simulink model "IdealFixedGearTransmissionSSC"  (R2026b)
settings: Solver=VariableStepAuto
undefined symbols (not defined in the file): Diff, Eng, PlntTransDampVect, Trans
libraries: fl_lib x6, nesl_utility x4, nesl_utility_internal x1, sdl_lib x1
settings Model: ModifiedByFormat=The MathWorks, Inc.  Creator=The MathWorks, Inc.  LastModifiedBy=The MathWorks, Inc.
settings OptimizationCC: ReuseModelBlockBuffer=off
settings DebuggingCC: SubsystemReferenceDiagnosticForUnitTest=warning
settings SimscapeCC: SimscapeUseEnergyAccounting=off

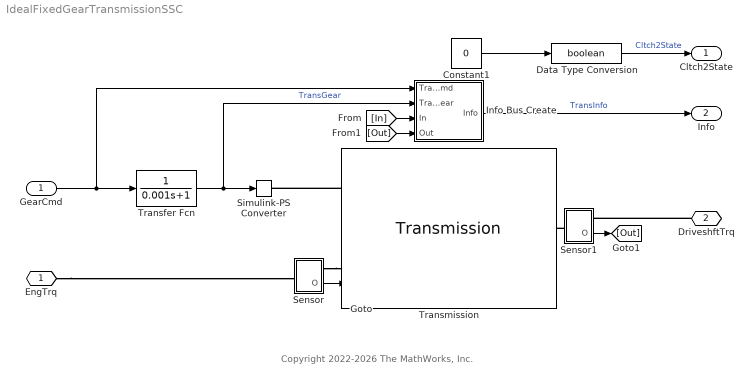
== system IdealFixedGearTransmissionSSC ==
  note: Copyright 2022-2026 The MathWorks, Inc.
  GearCmd : Inport
  Constant1 : Constant  Value=0  SampleTime=-1
  Data Type Conversion : DataTypeConversion  OutDataTypeStr=boolean  SaturateOnIntegerOverflow=off  RndMeth=Floor
  Info Bus Create : Subsystem
  Sensor : Subsystem
      settings: PortSchema="{\"entries\":[{\"content\":{\"sides\":[{\"content\":{\"connectorIds\":[\"LConn1\"]},\"type\":\"ConnectorPlacement.EquallySpacedRectSide\",\"uuid\":\"2e27b447-89d7-4d94-b9d2-8f612a4e25ed\"},{\"content\":{\"connectorIds\":[\"RConn1\",\"Out1\"],\"side\":\"RIGHT\"},\"type\":\"ConnectorPlacement.EquallySpacedRectSide\",\"uuid\":\"d649ff29-a00c-460e-9e09-fe3bc3dd9339\"},{\"content\":{\"side\":\"TOP\"},\"type\":\"ConnectorPlacement.EquallySpacedRectSide\",\"uuid\":\"c1caa1bf-44c8-4179-bd35-f8aecae525f1\"}]},\"type\":\"ConnectorPlacement.EquallySpacedConnector\",\"uuid\":\"741ea5ec-6556-46e5-ba1b-80e523f861d6\"}],\"packageUris\":[\"http://schema.mathworks.com/mf0/Connector/R2020b\"],\"version\":\"1.0\"}"
  Sensor1 : Subsystem
      settings: PortSchema="{\"entries\":[{\"content\":{\"sides\":[{\"content\":{\"connectorIds\":[\"LConn1\"]},\"type\":\"ConnectorPlacement.EquallySpacedRectSide\",\"uuid\":\"2e27b447-89d7-4d94-b9d2-8f612a4e25ed\"},{\"content\":{\"connectorIds\":[\"RConn1\",\"Out1\"],\"side\":\"RIGHT\"},\"type\":\"ConnectorPlacement.EquallySpacedRectSide\",\"uuid\":\"d649ff29-a00c-460e-9e09-fe3bc3dd9339\"},{\"content\":{\"side\":\"TOP\"},\"type\":\"ConnectorPlacement.EquallySpacedRectSide\",\"uuid\":\"c1caa1bf-44c8-4179-bd35-f8aecae525f1\"}]},\"type\":\"ConnectorPlacement.EquallySpacedConnector\",\"uuid\":\"741ea5ec-6556-46e5-ba1b-80e523f861d6\"}],\"packageUris\":[\"http://schema.mathworks.com/mf0/Connector/R2020b\"],\"version\":\"1.0\"}"
  Simulink-PS Converter : nesl_utility_internal/Simulink-PS Converter  PhysicalDomain=network_engine_domain  SubClassName=ps_input  LeftPortType=input  RightPortType=output  PseudoPeriodic=off  Frequencies=[]  NoiseDistribution=none  NoiseParameters=[]  Unit=1  AffineConversion=off  FilteringAndDerivatives=provide  SimscapeFilterOrder=1  InputFilterTimeConstant=0.001  UdotUserProvided=0
  Transfer Fcn : TransferFcn  Denominator=[0.001 1]
  Transmission : sdl_lib/Gears/Transmission  gear_ratios=PlntTransGearRatioVect(3:end)  reverse_ratio=PlntTransRvrseGearRatio  friction_model=sdl.enum.transmissionFriction.gear  efficiency=0.95  efficiency_tlu=PlntTransEffVect(3:end)  reverse_efficiency=PlntTransRvrseGearEff  pwr_thr=PlntTransPwrThresh W  kp=PlntTransStiff N*m/rad  kv=PlntTransDamp N*m*s/rad  initial_torque=PlntTransInitInTrq N*m  mu_visc=[PlntTransDampVect(2), PlntTransDampVect(2)] N*m*s/rad  t_friction=PlntTransCltchKinFricTrq N*m  t_locked=PlntTransCltchStatFricTrq N*m  shift_model=sdl.enum.transmissionShiftModel.instant  shift_time=PlntTransCltchShiftTime ms  w_tol=PlntTransCltchVelTol rad/s  initial_state_locked=sdl.enum.initial_lock.locked  thermal_port=simscape.enum.thermaleffects.omit  thermal_mass=100 kJ/K  initial_temperature=300 K
      settings: LogSimulationData=on
  EngTrq : PMIOPort  Side=Left
  DriveshftTrq : PMIOPort  Port=2  Side=Right
  Cltch2State : Outport  VectorParamsAs1DForOutWhenUnconnected=off
  Info : Outport  Port=2  VectorParamsAs1DForOutWhenUnconnected=off
  wires:
  Sensor1/1(O) -> [Out]
  Sensor/1(O) -> [In]
  Info Bus Create/1(Info) -> Info/1  "TransInfo"
  [Out] -> Info Bus Create/4(Out)
  [In] -> Info Bus Create/3(In)
  GearCmd/1 -> Transfer Fcn/1, Info Bus Create/1(TransGearCmd)
  Transfer Fcn/1 -> Simulink-PS Converter/1, Info Bus Create/2(TransGear)  "TransGear"
  Constant1/1 -> Data Type Conversion/1
  Data Type Conversion/1 -> Cltch2State/1  "Cltch2State"
  connections:
  Sensor1/LConn1 -- Transmission/RConn1
  Sensor/RConn1 -- Transmission/LConn2
  DriveshftTrq/RConn1 -- Sensor1/RConn1
  EngTrq/RConn1 -- Sensor/LConn1
  Transmission/LConn1 -- Simulink-PS Converter/RConn1

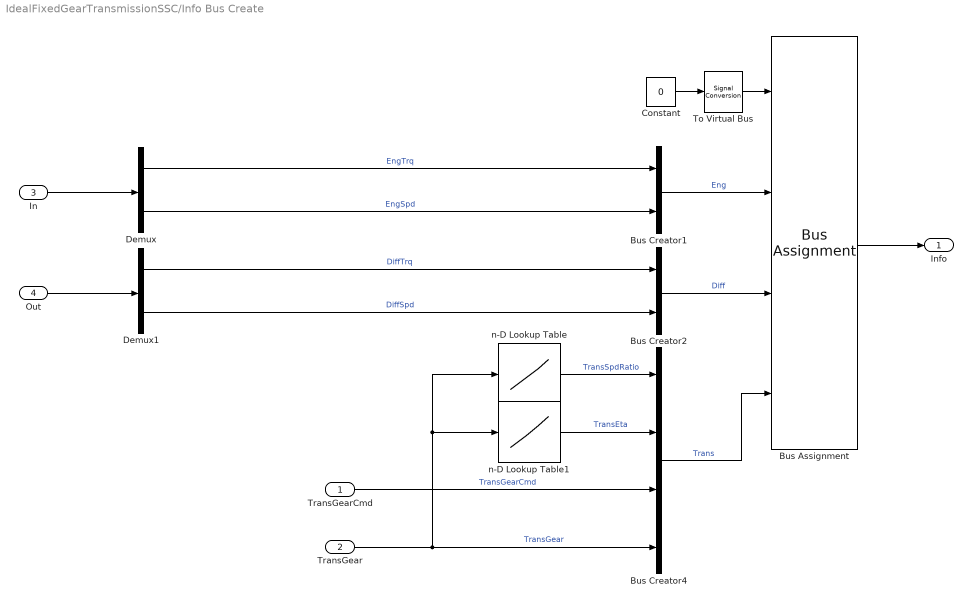
== system IdealFixedGearTransmissionSSC/Info Bus Create ==
  TransGearCmd : Inport
  TransGear : Inport  Port=2
  In : Inport  Port=3
  Out : Inport  Port=4
  Bus Assignment : BusAssignment  AssignedSignals=Eng,Diff,Trans
  Bus Creator1 : BusCreator  Inputs=2
  Bus Creator2 : BusCreator  Inputs=2
  Bus Creator4 : BusCreator  Inputs=4
  Constant : Constant  Value=0  OutDataTypeStr=Bus: InfoBUS  SampleTime=Inf
  Demux : Demux  Outputs=2
  Demux1 : Demux  Outputs=2
  To Virtual Bus : SignalConversion  ConversionOutput=Virtual bus  OverrideOpt=off
  n-D Lookup Table : Lookup_n-D  NumberOfTableDimensions=1  BreakpointsForDimension1=PlntTransGearNumVect(2:end)  BreakpointsForDimension3=[5, 7]  BeginIndexSearchUsingPreviousIndexResult=on  Table=PlntTransGearRatioVect(2:end)  InterpMethod=Nearest  ExtrapMethod=Clip  UseLastTableValue=on  InternalRulePriority=Speed  RndMeth=Simplest
  n-D Lookup Table1 : Lookup_n-D  NumberOfTableDimensions=1  BreakpointsForDimension1=PlntTransGearNumVect(2:end)  BreakpointsForDimension3=[5, 7]  BeginIndexSearchUsingPreviousIndexResult=on  Table=PlntTransEffVect(2:end)  InterpMethod=Nearest  ExtrapMethod=Clip  UseLastTableValue=on  InternalRulePriority=Speed  RndMeth=Simplest
  Info : Outport
  wires:
  To Virtual Bus/1 -> Bus Assignment/1
  Bus Assignment/1 -> Info/1
  Constant/1 -> To Virtual Bus/1
  Bus Creator2/1 -> Bus Assignment/3  "Diff"
  TransGear/1 -> Bus Creator4/4, n-D Lookup Table1/1, n-D Lookup Table/1  "TransGear"
  Demux/1 -> Bus Creator1/1  "EngTrq"
  n-D Lookup Table/1 -> Bus Creator4/1  "TransSpdRatio"
  Demux1/1 -> Bus Creator2/1  "DiffTrq"
  Demux/2 -> Bus Creator1/2  "EngSpd"
  Bus Creator1/1 -> Bus Assignment/2  "Eng"
  n-D Lookup Table1/1 -> Bus Creator4/2  "TransEta"
  Demux1/2 -> Bus Creator2/2  "DiffSpd"
  Bus Creator4/1 -> Bus Assignment/4  "Trans"
  In/1 -> Demux/1
  Out/1 -> Demux1/1
  TransGearCmd/1 -> Bus Creator4/3  "TransGearCmd"

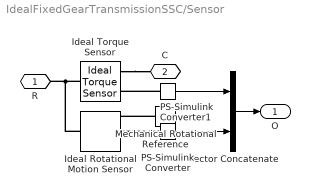
== system IdealFixedGearTransmissionSSC/Sensor ==
  Ideal Rotational Motion Sensor : fl_lib/Mechanical/Mechanical Sensors/Ideal Rotational Motion Sensor  reference=foundation.enum.MeasurementReference.difference  acceleration_port=false  velocity_port=true  position_port=true  wrap_angle=false  offset=0 rad
  Ideal Torque Sensor : fl_lib/Mechanical/Mechanical Sensors/Ideal Torque Sensor
  Mechanical Rotational Reference : fl_lib/Mechanical/Rotational Elements/Mechanical Rotational Reference
  PS-Simulink Converter : nesl_utility/PS-Simulink Converter  PhysicalDomain=network_engine_domain  SubClassName=ps_output  LeftPortType=input  RightPortType=output  PseudoPeriodic=off  Frequencies=[]  VectorFormat=inherit  Unit=inherit  AffineConversion=off
  PS-Simulink Converter1 : nesl_utility/PS-Simulink Converter  PhysicalDomain=network_engine_domain  SubClassName=ps_output  LeftPortType=input  RightPortType=output  PseudoPeriodic=off  Frequencies=[]  VectorFormat=inherit  Unit=inherit  AffineConversion=off
  Vector Concatenate : Concatenate
  R : PMIOPort  Side=Left
  C : PMIOPort  Port=2  Side=Right
  O : Outport
  wires:
  Vector Concatenate/1 -> O/1
  PS-Simulink Converter/1 -> Vector Concatenate/2
  PS-Simulink Converter1/1 -> Vector Concatenate/1
  connections:
  PS-Simulink Converter/LConn1 -- Ideal Rotational Motion Sensor/RConn2
  Mechanical Rotational Reference/LConn1 -- Ideal Rotational Motion Sensor/RConn1
  Ideal Torque Sensor/RConn1 -- C/RConn1
  Ideal Rotational Motion Sensor/LConn1 -- Ideal Torque Sensor/LConn1 -- R/RConn1
  PS-Simulink Converter1/LConn1 -- Ideal Torque Sensor/RConn2

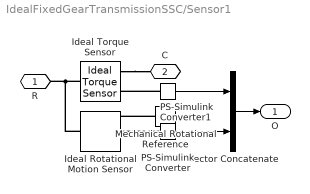
== system IdealFixedGearTransmissionSSC/Sensor1 ==
  Ideal Rotational Motion Sensor : fl_lib/Mechanical/Mechanical Sensors/Ideal Rotational Motion Sensor  reference=foundation.enum.MeasurementReference.difference  acceleration_port=false  velocity_port=true  position_port=true  wrap_angle=false  offset=0 rad
  Ideal Torque Sensor : fl_lib/Mechanical/Mechanical Sensors/Ideal Torque Sensor
  Mechanical Rotational Reference : fl_lib/Mechanical/Rotational Elements/Mechanical Rotational Reference
  PS-Simulink Converter : nesl_utility/PS-Simulink Converter  PhysicalDomain=network_engine_domain  SubClassName=ps_output  LeftPortType=input  RightPortType=output  PseudoPeriodic=off  Frequencies=[]  VectorFormat=inherit  Unit=inherit  AffineConversion=off
  PS-Simulink Converter1 : nesl_utility/PS-Simulink Converter  PhysicalDomain=network_engine_domain  SubClassName=ps_output  LeftPortType=input  RightPortType=output  PseudoPeriodic=off  Frequencies=[]  VectorFormat=inherit  Unit=inherit  AffineConversion=off
  Vector Concatenate : Concatenate
  R : PMIOPort  Side=Left
  C : PMIOPort  Port=2  Side=Right
  O : Outport
  wires:
  PS-Simulink Converter1/1 -> Vector Concatenate/1
  PS-Simulink Converter/1 -> Vector Concatenate/2
  Vector Concatenate/1 -> O/1
  connections:
  PS-Simulink Converter1/LConn1 -- Ideal Torque Sensor/RConn2
  R/RConn1 -- Ideal Torque Sensor/LConn1 -- Ideal Rotational Motion Sensor/LConn1
  Ideal Torque Sensor/RConn1 -- C/RConn1
  Mechanical Rotational Reference/LConn1 -- Ideal Rotational Motion Sensor/RConn1
  PS-Simulink Converter/LConn1 -- Ideal Rotational Motion Sensor/RConn2
